simulink model "simulation"  (R2017a)
settings: Solver=VariableStepAuto  StartTime=0.0  StopTime=2000  RelTol=1e-3  EnableMultiTasking=on
settings Model: Creator=DongHe  LastModifiedBy=Administrator
settings OptimizationCC: LifeSpan=inf
settings DebuggingCC: SFUnexpectedBacktrackingDiag=warning  SFNoUnconditionalDefaultTransitionDiag=warning  SFExecutionAtInitializationDiag=none
settings GRTTargetCC: TargetLangStandard=C89/C90 (ANSI)  GeneratePreprocessorConditionals=Disable all
settings ConfigComp: CovMetricSettings=dw  CovHtmlReporting=on  CovSaveCumulativeToWorkspaceVar=on  CovSaveSingleToWorkspaceVar=on  CovExternalEMLEnable=off

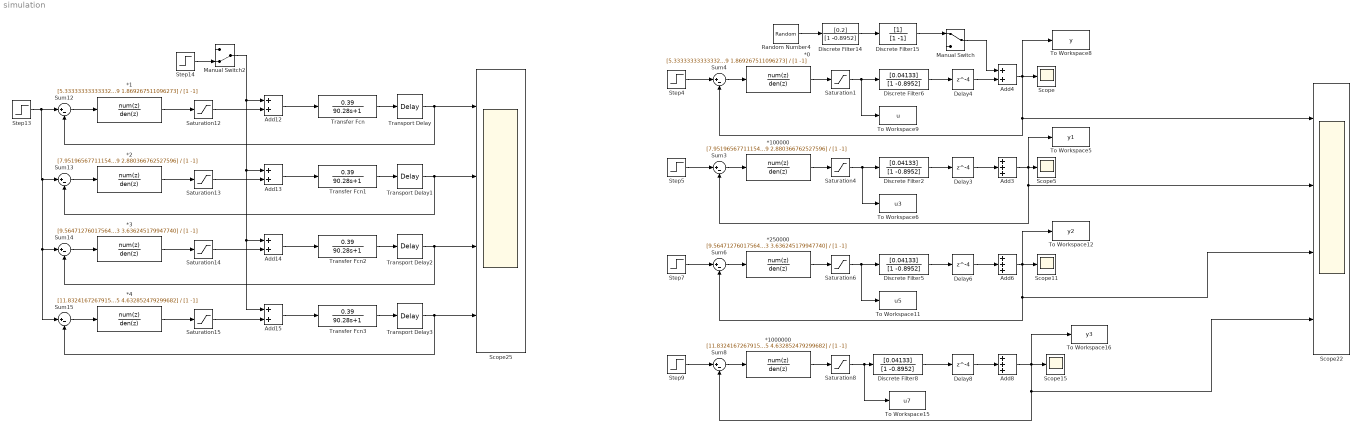
== system simulation ==
  *0 : DiscreteFilter  Numerator=[5.333333333333328 -6.875583654783349 1.869267511096273]  Denominator=[1 -1]  SampleTime=1
  *1 : DiscreteFilter  Numerator=[5.333333333333328 -6.875583654783349 1.869267511096273]  Denominator=[1 -1]  SampleTime=10
  *100000 : DiscreteFilter  Numerator=[7.951965677111540 -10.209895634199759 2.880366762527596]  Denominator=[1 -1]  SampleTime=1
  *1000000 : DiscreteFilter  Numerator=[11.832416726791548 -15.499283413672405 4.632852479299682]  Denominator=[1 -1]  SampleTime=1
  *2 : DiscreteFilter  Numerator=[7.951965677111540 -10.209895634199759 2.880366762527596]  Denominator=[1 -1]  SampleTime=10
  *250000 : DiscreteFilter  Numerator=[9.564712760175643 -12.416582123742563 3.636245179947740]  Denominator=[1 -1]  SampleTime=1
  *3 : DiscreteFilter  Numerator=[9.564712760175643 -12.416582123742563 3.636245179947740]  Denominator=[1 -1]  SampleTime=10
  *4 : DiscreteFilter  Numerator=[11.832416726791548 -15.499283413672405 4.632852479299682]  Denominator=[1 -1]  SampleTime=10
  Add{4,12..15} (5 alike) : Sum
  Add3 : Sum  Inputs=+++
  Add6 : Sum  Inputs=+++
  Add8 : Sum  Inputs=+++
  Delay{3..4,6,8} (4 alike) : Delay  DelayLength=4  SampleTime=1
  Discrete Filter14 : DiscreteFilter  Numerator=[0.2]  Denominator=[1 -0.8952]  SampleTime=1
  Discrete Filter15 : DiscreteFilter  Denominator=[1 -1]  SampleTime=1
  Discrete Filter{2,5..6,8} (4 alike) : DiscreteFilter  Numerator=[0.04133]  Denominator=[1 -0.8952]  SampleTime=1
  Manual Switch : ManualSwitch
  Manual Switch2 : ManualSwitch  CurrentSetting=0
  Random Number4 : RandomNumber  Variance=1e-5  SampleTime=1
  Saturation{1,4,6,8,12..15} (8 alike) : Saturate  UpperLimit=16  LowerLimit=0
  Scope{,5,11,15} (4 alike) : Scope
  Scope22 : Scope  NumInputPorts=4
  Scope25 : Scope  NumInputPorts=4
  Step13 : Step  Time=0  After=3  SampleTime=0
  Step14 : Step  Time=1000  SampleTime=0
  Step{4..5,7,9} (4 alike) : Step  Time=0  After=3  SampleTime=1
  Sum{3..4,6,8,12..15} (8 alike) : Sum  Inputs=|+-
  To Workspace11 : ToWorkspace  VariableName=u5  SaveFormat=Timeseries  SampleTime=-1
  To Workspace12 : ToWorkspace  VariableName=y2  SaveFormat=Timeseries  SampleTime=-1
  To Workspace15 : ToWorkspace  VariableName=u7  SaveFormat=Timeseries  SampleTime=-1
  To Workspace16 : ToWorkspace  VariableName=y3  SaveFormat=Timeseries  SampleTime=-1
  To Workspace5 : ToWorkspace  VariableName=y1  SaveFormat=Timeseries  SampleTime=-1
  To Workspace6 : ToWorkspace  VariableName=u3  SaveFormat=Timeseries  SampleTime=-1
  To Workspace8 : ToWorkspace  VariableName=y  SaveFormat=Timeseries  SampleTime=-1
  To Workspace9 : ToWorkspace  VariableName=u  SaveFormat=Timeseries  SampleTime=-1
  Transfer Fcn{,1..3} (4 alike) : TransferFcn  Numerator=[0.39]  Denominator=[90.28 1]
  Transport Delay{,1..3} (4 alike) : TransportDelay  DelayTime=31.98
  wires:
  Discrete Filter6/1 -> Delay4/1
  Delay4/1 -> Add4/2
  Step4/1 -> Sum4/1
  Sum4/1 -> *0/1
  *0/1 -> Saturation1/1
  Random Number4/1 -> Discrete Filter14/1
  Add4/1 -> Sum4/2, Scope22/1, Scope/1, To Workspace8/1
  Discrete Filter14/1 -> Discrete Filter15/1
  Discrete Filter15/1 -> Manual Switch/1
  Saturation1/1 -> To Workspace9/1, Discrete Filter6/1
  Discrete Filter2/1 -> Delay3/1
  Delay3/1 -> Add3/2
  Step5/1 -> Sum3/1
  Sum3/1 -> *100000/1
  *100000/1 -> Saturation4/1
  Add3/1 -> To Workspace5/1, Scope5/1, Sum3/2, Scope22/2
  Saturation4/1 -> To Workspace6/1, Discrete Filter2/1
  Discrete Filter5/1 -> Delay6/1
  Delay6/1 -> Add6/2
  Step7/1 -> Sum6/1
  Sum6/1 -> *250000/1
  *250000/1 -> Saturation6/1
  Add6/1 -> To Workspace12/1, Scope11/1, Scope22/3, Sum6/2
  Saturation6/1 -> To Workspace11/1, Discrete Filter5/1
  Discrete Filter8/1 -> Delay8/1
  Delay8/1 -> Add8/2
  Step9/1 -> Sum8/1
  Sum8/1 -> *1000000/1
  *1000000/1 -> Saturation8/1
  Add8/1 -> To Workspace16/1, Scope15/1, Scope22/4, Sum8/2
  Saturation8/1 -> To Workspace15/1, Discrete Filter8/1
  Manual Switch/1 -> Add4/1
  Saturation12/1 -> Add12/2
  Sum12/1 -> *1/1
  *1/1 -> Saturation12/1
  Transfer Fcn/1 -> Transport Delay/1
  Transport Delay/1 -> Sum12/2, Scope25/1
  Transport Delay1/1 -> Sum13/2, Scope25/2
  Transfer Fcn1/1 -> Transport Delay1/1
  Saturation13/1 -> Add13/2
  *2/1 -> Saturation13/1
  Sum13/1 -> *2/1
  Transport Delay2/1 -> Sum14/2, Scope25/3
  Transfer Fcn2/1 -> Transport Delay2/1
  Saturation14/1 -> Add14/2
  *3/1 -> Saturation14/1
  Sum14/1 -> *3/1
  Transport Delay3/1 -> Sum15/2, Scope25/4
  Transfer Fcn3/1 -> Transport Delay3/1
  Step13/1 -> Sum15/1, Sum14/1, Sum13/1, Sum12/1
  Saturation15/1 -> Add15/2
  *4/1 -> Saturation15/1
  Sum15/1 -> *4/1
  Add12/1 -> Transfer Fcn/1
  Add13/1 -> Transfer Fcn1/1
  Add14/1 -> Transfer Fcn2/1
  Add15/1 -> Transfer Fcn3/1
  Step14/1 -> Manual Switch2/2
  Manual Switch2/1 -> Add15/1, Add14/1, Add13/1, Add12/1
